simulink model "simlink1"  (R2017b)
settings: Solver=VariableStepAuto  StartTime=0.0  StopTime=20  RelTol=1e-3
libraries: simulink x3
settings Model: Creator=Administrator  LastModifiedBy=Administrator

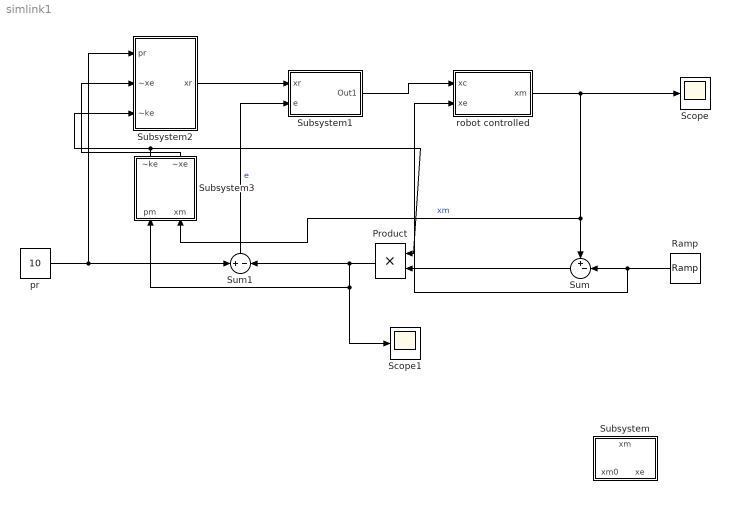
== system simlink1 ==
  Product : Product
  Ramp : simulink/Sources/Ramp  slope=0.5  start=4  X0=0.6
  Scope : Scope
  Scope1 : Scope
  Subsystem : Subsystem
  Subsystem1 : Subsystem
  Subsystem2 : Subsystem
  Subsystem3 : Subsystem
  Sum : Sum  Inputs=+-|
  Sum1 : Sum  Inputs=+|-
  pr : Constant  Value=10
  robot controlled : Subsystem
  wires:
  Subsystem3/1(~ke) -> Product/1, Subsystem2/3(~ke)
  pr/1 -> Subsystem2/1(pr), Sum1/1
  Subsystem3/2(~xe) -> Subsystem2/2(~xe)
  Sum1/1 -> Subsystem1/2(e)  "e"
  Subsystem2/1(xr) -> Subsystem1/1(xr)
  Subsystem1/1(Out1) -> robot controlled/1(xc)
  Product/1 -> Scope1/1, Subsystem3/1(pm), Sum1/2
  Sum/1 -> Product/2
  robot controlled/1("xm ") -> Subsystem3/2(xm), Sum/1, Scope/1  "xm"
  Ramp/1 -> robot controlled/2(xe), Sum/2

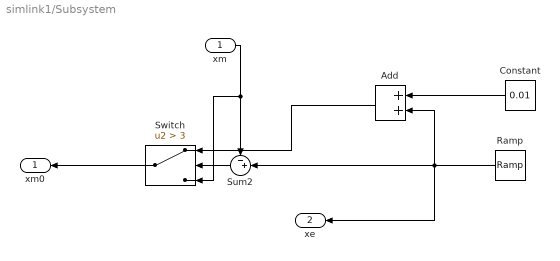
== system simlink1/Subsystem ==
  xm : Inport
  Add : Sum
  Constant : Constant  Value=0.01
  Ramp : simulink/Sources/Ramp  slope=1  start=3  X0=10
  Sum2 : Sum  Inputs=-+|
  Switch : Switch  Criteria=u2 > Threshold  Threshold=3
  xm0 : Outport
  xe : Outport  Port=2
  wires:
  xm/1 -> Switch/3, Sum2/1
  Ramp/1 -> Sum2/2, xe/1, Add/2
  Switch/1 -> xm0/1
  Sum2/1 -> Switch/2
  Constant/1 -> Add/1
  Add/1 -> Switch/1

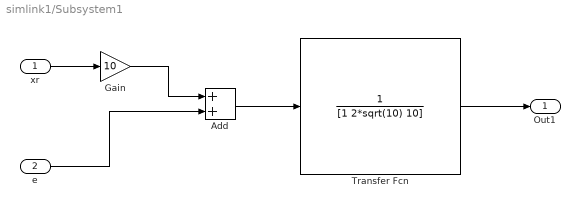
== system simlink1/Subsystem1 ==
  xr : Inport
  e : Inport  Port=2
  Add : Sum
  Gain : Gain  Gain=10
  Transfer Fcn : TransferFcn  Denominator=[1 2*sqrt(10) 10]
  Out1 : Outport
  wires:
  xr/1 -> Gain/1
  Gain/1 -> Add/1
  e/1 -> Add/2
  Add/1 -> Transfer Fcn/1
  Transfer Fcn/1 -> Out1/1

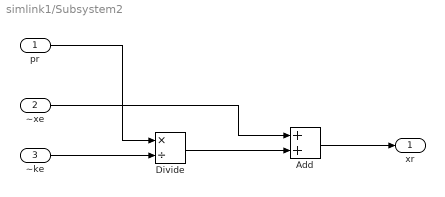
== system simlink1/Subsystem2 ==
  pr : Inport
  ~xe : Inport  Port=2
  ~ke : Inport  Port=3
  Add : Sum
  Divide : Product  Inputs=*/
  xr : Outport
  wires:
  pr/1 -> Divide/1
  ~ke/1 -> Divide/2
  ~xe/1 -> Add/1
  Divide/1 -> Add/2
  Add/1 -> xr/1

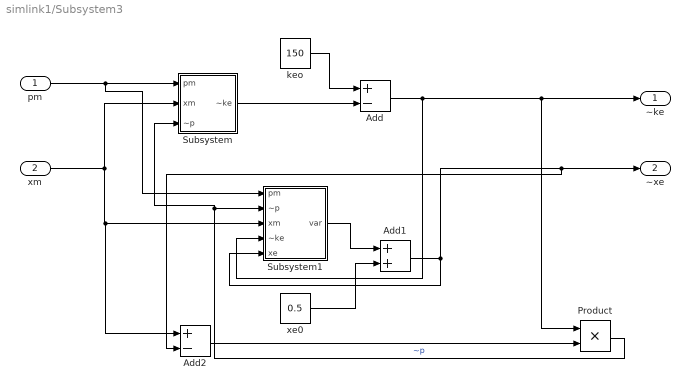
== system simlink1/Subsystem3 ==
  pm : Inport
  xm : Inport  Port=2
  Add : Sum  Inputs=+-
  Add1 : Sum
  Add2 : Sum  Inputs=+-
  Product : Product
  Subsystem : Subsystem
  Subsystem1 : Subsystem
  keo : Constant  Value=150
  xe0 : Constant  Value=0.5
  ~ke : Outport
  ~xe : Outport  Port=2
  wires:
  pm/1 -> Subsystem1/1(pm), Subsystem/1(pm)
  xm/1 -> Subsystem/2(xm), Add2/1, Subsystem1/3(xm)
  keo/1 -> Add/1
  Add/1 -> Subsystem1/4(~ke), Product/1, ~ke/1
  Subsystem/1(~ke) -> Add/2
  Subsystem1/1(var) -> Add1/1
  xe0/1 -> Add1/2
  Add1/1 -> Subsystem1/5("xe "), Add2/2, ~xe/1
  Add2/1 -> Product/2
  Product/1 -> Subsystem/3(~p), Subsystem1/2(~p)  "~p"

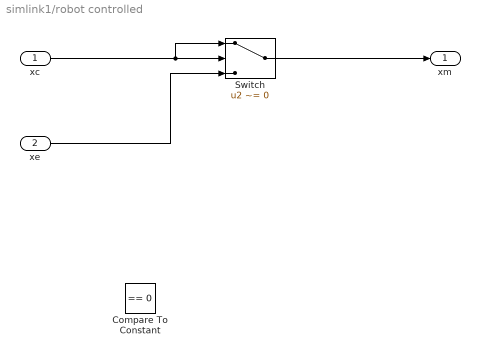
== system simlink1/robot controlled ==
  xc : Inport
  xe : Inport  Port=2
  Compare To Constant : simulink/Logic and Bit Operations/Compare To Constant  relop===  const=0  OutDataTypeStr=boolean
  Switch : Switch  Criteria=u2 ~= 0  Threshold=0.2
  "xm " : Outport
  wires:
  Switch/1 -> "xm "/1
  xc/1 -> Switch/1, Switch/2
  xe/1 -> Switch/3

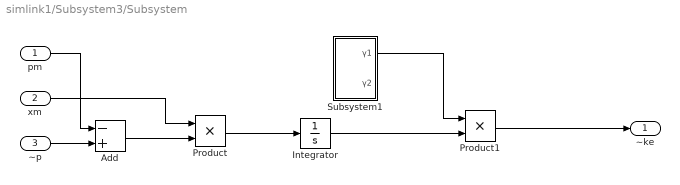
== system simlink1/Subsystem3/Subsystem ==
  pm : Inport
  xm : Inport  Port=2
  ~p : Inport  Port=3
  Add : Sum  Inputs=-+
  Integrator : Integrator
  Product : Product
  Product1 : Product
  Subsystem1 : Subsystem
  ~ke : Outport
  wires:
  ~p/1 -> Add/2
  pm/1 -> Add/1
  xm/1 -> Product/1
  Add/1 -> Product/2
  Product/1 -> Integrator/1
  Integrator/1 -> Product1/2
  Product1/1 -> ~ke/1
  Subsystem1/1(γ1) -> Product1/1

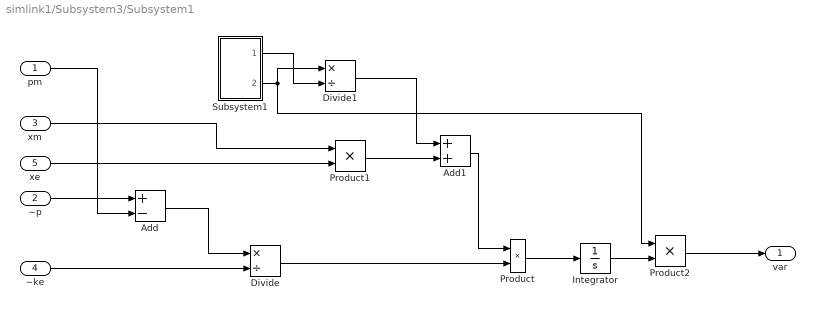
== system simlink1/Subsystem3/Subsystem1 ==
  pm : Inport
  ~p : Inport  Port=2
  xm : Inport  Port=3
  ~ke : Inport  Port=4
  "xe " : Inport  Port=5
  Add : Sum  Inputs=+-
  Add1 : Sum
  Divide : Product  Inputs=*/
  Divide1 : Product  Inputs=*/
  Integrator : Integrator
  Product : Product
  Product1 : Product
  Product2 : Product
  Subsystem1 : Subsystem
  var : Outport
  wires:
  pm/1 -> Add/2
  ~p/1 -> Add/1
  Add/1 -> Divide/1
  ~ke/1 -> Divide/2
  Divide/1 -> Product/2
  xm/1 -> Product1/1
  Divide1/1 -> Add1/1
  Product1/1 -> Add1/2
  Add1/1 -> Product/1
  Integrator/1 -> Product2/2
  Product2/1 -> var/1
  "xe "/1 -> Product1/2
  Product/1 -> Integrator/1
  Subsystem1/1(gama1) -> Divide1/2
  Subsystem1/2(gama2) -> Product2/1, Divide1/1

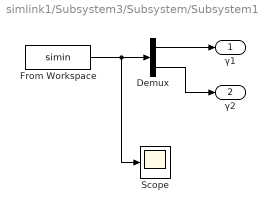
== system simlink1/Subsystem3/Subsystem/Subsystem1 ==
  Demux : Demux  Outputs=2
  From Workspace : FromWorkspace  VariableName=simin  SampleTime=0
  Scope : Scope
  γ1 : Outport
  γ2 : Outport  Port=2
  wires:
  Demux/2 -> γ2/1
  Demux/1 -> γ1/1
  From Workspace/1 -> Scope/1, Demux/1

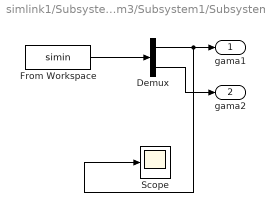
== system simlink1/Subsystem3/Subsystem1/Subsystem1 ==
  Demux : Demux  Outputs=2
  From Workspace : FromWorkspace  VariableName=simin  SampleTime=0
  Scope : Scope
  gama1 : Outport
  gama2 : Outport  Port=2
  wires:
  Demux/2 -> gama2/1
  Demux/1 -> Scope/1, gama1/1
  From Workspace/1 -> Demux/1
